simulink model "TRUAV_Dynamics_from_GTRS_trim"  (R2022b)
settings: Solver=ode4  StartTime=0.0  StopTime=3  FixedStep=0.004  RelTol=1e-3
values from neighbouring files (symbols this model uses):
  a_sound = 1116.45    [init_0_GTRS_data_Run_this_file.m]
  alpha_F_rad = alpha_F_deg * (pi/180)    [init_Vetical_2_Table.m]
  alpha_F_rad_table = alpha_F_table * (pi/180)    [init_Fuselage_Aero_Table.m]
  alpha_H_rad = alpha_H_deg * (pi/180)    [init_Horizontal_Table.m]
  alpha_HD_rad = alpha_HD_deg * (pi/180)    [init_Horizontal_C_D_Table.m]
  alpha_r0 = 0    [init_0_GTRS_data_Run_this_file.m]
  alpha_WF_epsilon_M_rad = alpha_WF_deg * pi/180    [init_WingWake_Deflection_Table.m]
  alpha_WS_CL_rad = alpha_WS_CL_deg * (pi/180)    [init_Wing_Slide_Table.m]
  b_w = 32.17    [init_0_GTRS_data_Run_this_file.m]
  beta_F_rad = beta_F_deg * (pi/180)    [init_Vetical_2_Table.m]
  beta_LD_rad_table = beta_LD_table * (pi/180)    [init_Fuselage_Aero_Table.m]
  beta_m_epsilon_M_rad = beta_m_deg * pi/180    [init_WingWake_Deflection_Table.m]
  beta_m_rad_cn = beta_m_deg_cn * pi/180    [init_Wing_Free_Table.m]
  beta_M_rad_table = beta_M_table  * (pi/180)    [init_Fuselage_Aero_Table.m]
  beta_m_S_rad = beta_m_S_deg * (pi/180)    [init_Vetical_2_Table.m]
  beta_m_WS_CL_rad = beta_m_WS_CL_deg * (pi/180)    [init_Wing_Slide_Table.m]
  beta_rad_brk = beta_KBR_rad    [init_Vetical_2_Table.m]
  beta_v_rad = beta_v_deg * (pi/180)    [init_Vetical_1_Table.m]
  beta_vD_rad = beta_vD_deg * (pi/180)    [init_Vetical_1_Table.m]
  beta_WF_Cl_rad = beta_W_deg * (pi/180)    [init_Wing_Free_Table.m]
  beta_WF_CL_rad = beta_CL_deg * (pi/180)    [init_Wing_Free_Table.m]
  beta_YlN_rad_table = beta_YlN_table * (pi/180)    [init_Fuselage_Aero_Table.m]
  c_HW = 3.92    [init_0_GTRS_data_Run_this_file.m]
  C_l_beta_CLwp_table = [ ... (first row only)    [init_Wing_Free_Table.m]
  C_l_beta_pro_CLwp_table = [ ... (first row only)    [init_Wing_Free_Table.m]
  C_L_delta_a_table = [0.00316, 0.00396, 0.00476, 0]    [init_Wing_Free_Table.m]
  C_LHB = -0.00422    [init_0_GTRS_data_Run_this_file.m]
  C_lp_C_LWP = -0.774    [init_0_GTRS_data_Run_this_file.m]
  C_m_wp_table = [ ... (first row only)    [init_Wing_Free_Table.m]
  C_MHA = 0    [init_0_GTRS_data_Run_this_file.m]
  C_MHO = 0    [init_0_GTRS_data_Run_this_file.m]
  c_R = 14/12    (= 1.16666666667)    [init_0_GTRS_data_Run_this_file.m]
  c_w = 5.225    [init_0_GTRS_data_Run_this_file.m]
  C_Y_beta = 0    [init_0_GTRS_data_Run_this_file.m]
  CD0_high_Mach_data = [0.0177, 0.0178, 0.0179, 0.0405]    [init_Wing_Free_Table.m]
  CD_4D_table = zeros(49, 4, 2, 4)    [init_Wing_Slide_Table.m]
  CDH_2D_table = zeros(length(alpha_HD_deg), length(mach_vec))    [init_Horizontal_C_D_Table.m]
  CDV_2D_table = zeros(length(beta_vD_deg), length(mach_vec))    [init_Vetical_1_Table.m]
  CL_4D_table = zeros(49, 4, 2, 4)    [init_Wing_Slide_Table.m]
  CLH_3D_table = zeros(length(alpha_H_deg), length(delta_e_deg), length(mach_vec))    [init_Horizontal_Table.m]
  CYV_3D_table = zeros(length(beta_v_deg), length(delta_r_deg), length(mach_vec))    [init_Vetical_1_Table.m]
  D_alpha_table = [D_part1, D_part2, D_part3, D_part4]    [init_Fuselage_Aero_Table.m]
  D_beta_table = [ fliplr(D_beta_half(2:end)),  D_beta_half]    [init_Fuselage_Aero_Table.m]
  D_ke = 0.24    [init_0_GTRS_data_Run_this_file.m]
  D_Kr = 0.24    [init_0_GTRS_data_Run_this_file.m]    (also in init_Vetical_1_Table.m)
  DBFO = -1.56    [init_0_GTRS_data_Run_this_file.m]
  delta_e_rad = delta_e_deg * (pi/180)    [init_Horizontal_Table.m]
  delta_r_deg = [-20, -15, 0, 15, 20]    [init_Vetical_1_Table.m]
  DLANG = -0.5    [init_0_GTRS_data_Run_this_file.m]
  epsilon_W_table = permute(epsilon_W_3D, [3, 1, 2])    [init_WingWake_Deflection_Table.m]
  flap_rad = flap_deg * (pi/180)    [init_Wing_Free_Table.m]    (also in init_Wing_Slide_Table.m)
  ft2m = 0.3048    [init_0_GTRS_data_Run_this_file.m]
  h_HW = [-0.5838, 0.01158, 0.5967, 0.002547,-2.2519]    [init_0_GTRS_data_Run_this_file.m]
  I_b = 102.5    [init_0_GTRS_data_Run_this_file.m]
  i_H = 0    [init_0_GTRS_data_Run_this_file.m]
  i_v = 0    [init_0_GTRS_data_Run_this_file.m]
  i_w = 0    [init_0_GTRS_data_Run_this_file.m]
  in2ft = 1/12    (= 0.0833333333333)    [init_0_GTRS_data_Run_this_file.m]
  Ixx = 52795    [init_0_GTRS_data_Run_this_file.m]
  Ixz = 1234    [init_0_GTRS_data_Run_this_file.m]
  Iyy = 21360    [init_0_GTRS_data_Run_this_file.m]
  Izz = 66335    [init_0_GTRS_data_Run_this_file.m]
  K1delta_data = [ ... (first row only)    [init_Wing_Free_Table.m]
  K_coeffs = [1.6 0]    [init_0_GTRS_data_Run_this_file.m]
  K_FWDF = -0.0035    [init_0_GTRS_data_Run_this_file.m]
  K_FWO = 1.4    [init_0_GTRS_data_Run_this_file.m]
  K_HNU = 0.8    [init_0_GTRS_data_Run_this_file.m]
  K_vNU = 1    [init_Vetical_1_Table.m]
  KBR_table = KBR_table_full    [init_Vetical_2_Table.m]
  Kn_delta_data = [ ... (first row only)    [init_Wing_Free_Table.m]
  Kno_delta_data = [ ... (first row only)    [init_Wing_Free_Table.m]
  L_alpha_table = [L_part1, L_part2, L_part3, L_part4]    [init_Fuselage_Aero_Table.m]
  L_beta_table = [ fliplr(L_beta_half(2:end)),  L_beta_half]    [init_Fuselage_Aero_Table.m]
  l_beta_table = [l_beta_neg, l_beta_pos]    [init_Fuselage_Aero_Table.m]
  L_n = 4.667    [init_0_GTRS_data_Run_this_file.m]
  lambda_w = -6.5*deg2rad    (= -0.11344640138)    [init_0_GTRS_data_Run_this_file.m]
  LBFO = -7.23    [init_0_GTRS_data_Run_this_file.m]
  LLANG = 0    [init_0_GTRS_data_Run_this_file.m]
  m2ft = 1/ft2m    (= 3.28083989501)    [init_0_GTRS_data_Run_this_file.m]
  M_alpha_table = [M_part1, M_part2, M_part3, M_part4]    [init_Fuselage_Aero_Table.m]
  M_beta_table = [ fliplr(M_beta_half(2:end)), M_beta_half]    [init_Fuselage_Aero_Table.m]
  Mach_brk = [0.2, 0.4, 0.5, 0.6]    [init_Wing_Free_Table.m]
  mach_vec = [0.2, 0.4, 0.5, 0.6]    [init_Horizontal_C_D_Table.m]    (also in init_Horizontal_Table.m; init_Vetical_1_Table.m)
  mass = 403.7    [init_0_GTRS_data_Run_this_file.m]
  mast_rad = mast_deg * pi/180    [init_Wing_Free_Table.m]
  MBFO = 66.5    [init_0_GTRS_data_Run_this_file.m]
  Mn_X_ke = [0 0.2 0.4 0.5 0.6 0.7]    [init_Horizontal_Table.m]
  N_beta_table = [N_beta_neg, N_beta_pos]    [init_Fuselage_Aero_Table.m]
  pos_x_CG = 300    [init_0_GTRS_data_Run_this_file.m]
  pos_x_H = 300    [init_0_GTRS_data_Run_this_file.m]
  pos_x_HW = 560    [init_0_GTRS_data_Run_this_file.m]
  pos_x_Nac = 291.7    [init_0_GTRS_data_Run_this_file.m]
  pos_x_V = 570    [init_0_GTRS_data_Run_this_file.m]
  pos_x_W = 291.7    [init_0_GTRS_data_Run_this_file.m]
  pos_y_CG = 0    [init_0_GTRS_data_Run_this_file.m]
  pos_y_H = 193    [init_0_GTRS_data_Run_this_file.m]
  pos_y_HW = 0    [init_0_GTRS_data_Run_this_file.m]
  pos_y_Nac = 193    [init_0_GTRS_data_Run_this_file.m]
  pos_y_V = 115.69    [init_0_GTRS_data_Run_this_file.m]
  pos_y_W = 96.6    [init_0_GTRS_data_Run_this_file.m]
  pos_z_CG = 81.65    [init_0_GTRS_data_Run_this_file.m]
  pos_z_H = 100    [init_0_GTRS_data_Run_this_file.m]
  pos_z_HW = 103    [init_0_GTRS_data_Run_this_file.m]
  pos_z_Nac = 118    [init_0_GTRS_data_Run_this_file.m]
  pos_z_V = 77    [init_0_GTRS_data_Run_this_file.m]
  pos_z_W = 96    [init_0_GTRS_data_Run_this_file.m]
  R = 12.5    [init_0_GTRS_data_Run_this_file.m]
  rho = 0.002376    [init_0_GTRS_data_Run_this_file.m]
  s_HW = 50.25    [init_0_GTRS_data_Run_this_file.m]
  S_max = 56    [init_0_GTRS_data_Run_this_file.m]
  S_v = 20.25    [init_0_GTRS_data_Run_this_file.m]
  S_w = 181    [init_0_GTRS_data_Run_this_file.m]
  Sidewash_4D = zeros(length(alpha_F_deg), length(beta_F_deg), length(beta_m_S_deg), length(delta_F_S_deg))    [init_Vetical_2_Table.m]
  slugft2kgm = 1.35582    [init_0_GTRS_data_Run_this_file.m]
  tau_e = 0.518    [init_0_GTRS_data_Run_this_file.m]
  tau_r = 0.27    [init_0_GTRS_data_Run_this_file.m]    (also in init_Vetical_1_Table.m)
  theta_0_R = 0.750    (= 0.75)    [init_0_GTRS_data_Run_this_file.m]
  theta_0_W = 1.187    [init_0_GTRS_data_Run_this_file.m]
  theta_twist = -41*deg2rad    (= -0.715584993318)    [init_0_GTRS_data_Run_this_file.m]
  u_max = 1181/12    (= 98.4166666667)    [init_0_GTRS_data_Run_this_file.m]
  ... (+3 more)
undefined symbols (not defined in the file or in its folder): beta_m_rad, F, Light, MIL, sigbuilder_block, tilt_cmd
libraries: simulink x2, sharedtransform x2, aerolibasang x2, aerolibwind2 x1
(part 2 of 4)

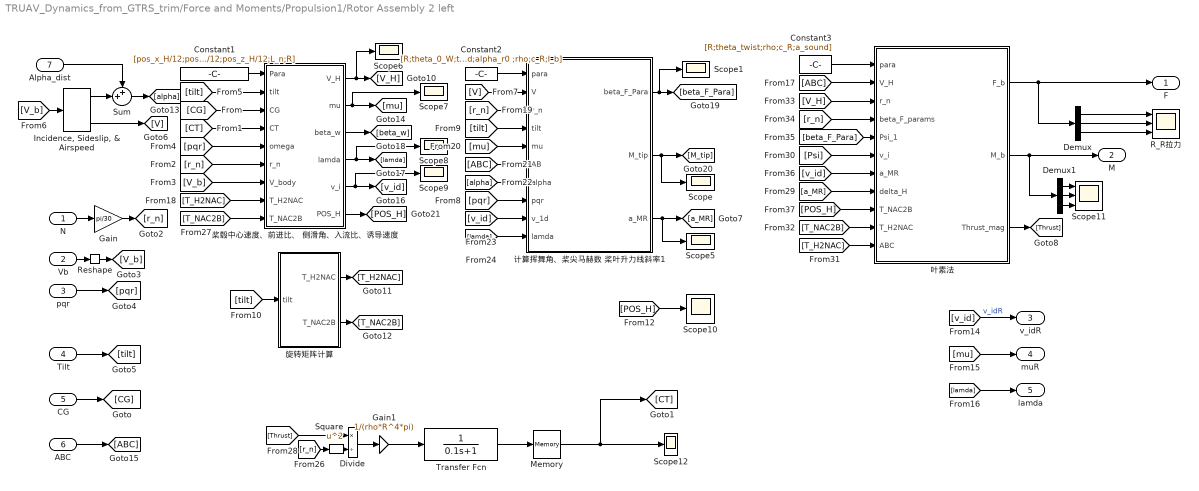
== system TRUAV_Dynamics_from_GTRS_trim/Force and Moments/Propulsion1/Rotor Assembly 2 left ==
  N : Inport
  Vb : Inport  Port=2
  pqr : Inport  Port=3
  Tilt : Inport  Port=4
  CG : Inport  Port=5
  ABC : Inport  Port=6
  Alpha_dist : Inport  Port=7
  Constant1 : Constant  Value=[pos_x_H/12;pos_y_H/12;pos_z_H/12;L_n;R]
  Constant2 : Constant  Value=[R;theta_0_W;theta_0_R;theta_twist;a_sound;alpha_r0 ;rho;c_R;I_b]
  Constant3 : Constant  Value=[R;theta_twist;rho;c_R;a_sound]
  Demux : Demux  Outputs=3
  Demux1 : Demux  Outputs=3
  Divide : Product  Inputs=*/
  Gain : Gain  Gain=pi/30
  Gain1 : Gain  Gain=1/(rho*R^4*pi)
  "Incidence, Sideslip, & Airspeed" : aerolibasang/Incidence, Sideslip, & Airspeed
  Memory : Memory  InitialCondition=0.02
  R_R拉力 : Scope  NumInputPorts=3
  Reshape : Reshape  OutputDimensionality=Column vector (2-D)
  Scope{,1,5..10,12} (9 alike) : Scope
  Scope11 : Scope  NumInputPorts=3
  Square : Math  Operator=square
  Sum : Sum  Inputs=++|
  Transfer Fcn : TransferFcn  Denominator=[0.1 1]
  叶素法 : MATLAB Function  TreatAsAtomicUnit=on
  旋转矩阵计算 : MATLAB Function  TreatAsAtomicUnit=on
  桨毂中心速度、前进比、 侧滑角、入流比、诱导速度 : MATLAB Function  TreatAsAtomicUnit=on
  计算挥舞角、桨尖马赫数 桨叶升力线斜率1 : MATLAB Function  TreatAsAtomicUnit=on
  F : Outport
  M : Outport  Port=2
  v_idR : Outport  Port=3
  muR : Outport  Port=4
  lamda : Outport  Port=5
  wires:
  Demux1/3 -> Scope11/3
  Demux1/2 -> Scope11/2
  Demux1/1 -> Scope11/1
  Demux/3 -> R_R拉力/3
  Demux/2 -> R_R拉力/2
  Demux/1 -> R_R拉力/1
  [Psi] -> 叶素法/6(v_i)
  桨毂中心速度、前进比、 侧滑角、入流比、诱导速度/3(beta_w) -> [beta_w]
  Reshape/1 -> [V_b]
  [POS_H] -> Scope10/1
  [T_NAC2B] -> 桨毂中心速度、前进比、 侧滑角、入流比、诱导速度/9(T_NAC2B)
  Gain/1 -> [r_n]
  pqr/1 -> [pqr]
  N/1 -> Gain/1
  Constant1/1 -> 桨毂中心速度、前进比、 侧滑角、入流比、诱导速度/1(Para)
  CG/1 -> [CG]
  [CG] -> 桨毂中心速度、前进比、 侧滑角、入流比、诱导速度/3(CG)
  [CT] -> 桨毂中心速度、前进比、 侧滑角、入流比、诱导速度/4(CT)
  [r_n] -> 桨毂中心速度、前进比、 侧滑角、入流比、诱导速度/6(r_n)
  Vb/1 -> Reshape/1
  [V_b] -> 桨毂中心速度、前进比、 侧滑角、入流比、诱导速度/7(V_body)
  [pqr] -> 桨毂中心速度、前进比、 侧滑角、入流比、诱导速度/5(omega)
  Tilt/1 -> [tilt]
  [tilt] -> 桨毂中心速度、前进比、 侧滑角、入流比、诱导速度/2(tilt)
  [V] -> 计算挥舞角、桨尖马赫数 桨叶升力线斜率1/2(V)
  [tilt] -> 计算挥舞角、桨尖马赫数 桨叶升力线斜率1/4(tilt)
  Constant2/1 -> 计算挥舞角、桨尖马赫数 桨叶升力线斜率1/1(para)
  计算挥舞角、桨尖马赫数 桨叶升力线斜率1/3(a_MR) -> [a_MR], Scope5/1
  [pqr] -> 计算挥舞角、桨尖马赫数 桨叶升力线斜率1/8(pqr)
  桨毂中心速度、前进比、 侧滑角、入流比、诱导速度/1(V_H) -> [V_H], Scope6/1
  [tilt] -> 旋转矩阵计算/1(tilt)
  旋转矩阵计算/1(T_H2NAC) -> [T_H2NAC]
  旋转矩阵计算/2(T_NAC2B) -> [T_NAC2B]
  [T_H2NAC] -> 桨毂中心速度、前进比、 侧滑角、入流比、诱导速度/8(T_H2NAC)
  桨毂中心速度、前进比、 侧滑角、入流比、诱导速度/2(mu) -> [mu], Scope7/1
  [r_n] -> 计算挥舞角、桨尖马赫数 桨叶升力线斜率1/3(r_n)
  [mu] -> 计算挥舞角、桨尖马赫数 桨叶升力线斜率1/5(mu)
  [ABC] -> 计算挥舞角、桨尖马赫数 桨叶升力线斜率1/6(AB)
  [alpha] -> 计算挥舞角、桨尖马赫数 桨叶升力线斜率1/7(alpha)
  桨毂中心速度、前进比、 侧滑角、入流比、诱导速度/5(v_i) -> [v_id], Scope9/1
  [v_id] -> 计算挥舞角、桨尖马赫数 桨叶升力线斜率1/9(v_1d)
  桨毂中心速度、前进比、 侧滑角、入流比、诱导速度/4(lamda) -> [lamda], Scope8/1
  [lamda] -> 计算挥舞角、桨尖马赫数 桨叶升力线斜率1/10(lamda)
  计算挥舞角、桨尖马赫数 桨叶升力线斜率1/1(beta_F_Para) -> [beta_F_Para], Scope1/1
  计算挥舞角、桨尖马赫数 桨叶升力线斜率1/2(M_tip) -> [M_tip], Scope/1
  桨毂中心速度、前进比、 侧滑角、入流比、诱导速度/6(POS_H) -> [POS_H]
  ABC/1 -> [ABC]
  [POS_H] -> 叶素法/9(T_NAC2B)
  [v_id] -> 叶素法/7(a_MR)
  [beta_F_Para] -> 叶素法/5(Psi_1)
  [r_n] -> 叶素法/4(beta_F_params)
  [V_H] -> 叶素法/3(r_n)
  Constant3/1 -> 叶素法/1(para)
  [a_MR] -> 叶素法/8(delta_H)
  [T_NAC2B] -> 叶素法/10(T_H2NAC)
  [T_H2NAC] -> 叶素法/11(ABC)
  [v_id] -> v_idR/1  "v_idR"
  [lamda] -> lamda/1
  [mu] -> muR/1
  [ABC] -> 叶素法/2(V_H)
  叶素法/1(F_b) -> F/1, Demux/1
  [r_n] -> Square/1
  Transfer Fcn/1 -> Memory/1
  [Thrust] -> Divide/1
  Divide/1 -> Gain1/1
  Square/1 -> Divide/2
  Gain1/1 -> Transfer Fcn/1
  叶素法/3(Thrust_mag) -> [Thrust]
  Memory/1 -> [CT], Scope12/1
  [V_b] -> "Incidence, Sideslip, & Airspeed"/1
  Alpha_dist/1 -> Sum/1
  Sum/1 -> [alpha]
  "Incidence, Sideslip, & Airspeed"/1 -> Sum/2
  "Incidence, Sideslip, & Airspeed"/3 -> [V]
  叶素法/2(M_b) -> Demux1/1, M/1

== system TRUAV_Dynamics_from_GTRS_trim/Force and Moments/Propulsion1/Tilt Servo Dynamics ==
  TiltA : Inport
  Tilt1 : Outport
  wires:
  TiltA/1 -> Tilt1/1  "Tilt1"

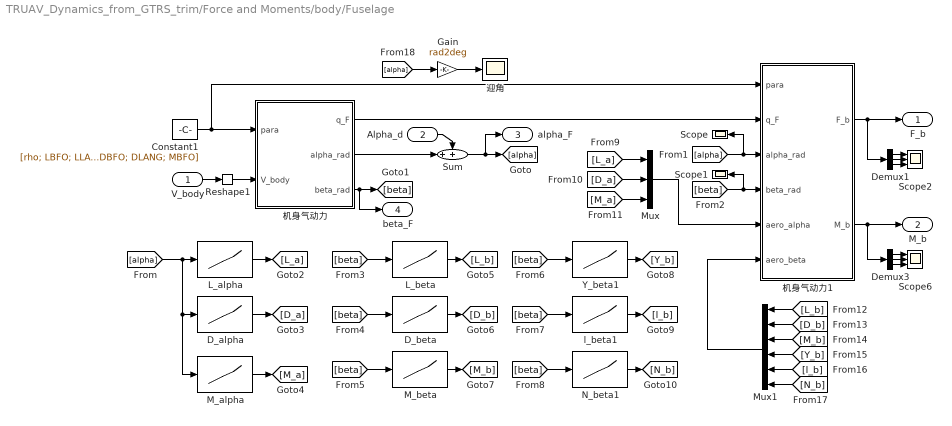
== system TRUAV_Dynamics_from_GTRS_trim/Force and Moments/body/Fuselage ==
  V_body : Inport
  Alpha_d : Inport  Port=2
  Constant1 : Constant  Value=[rho; LBFO; LLANG; DBFO; DLANG; MBFO]
  D_alpha : Lookup_n-D  NumberOfTableDimensions=1  LookupTableObject=''  BreakpointsForDimension1=alpha_F_rad_table  BreakpointsForDimension1FirstPoint=10  BreakpointsForDimension2FirstPoint=10  BreakpointsForDimension1Spacing=12  BreakpointsForDimension2Spacing=12  Table=D_alpha_table  DiagnosticForOutOfRangeInput=Error  InternalRulePriority=Speed  RndMeth=Simplest
  D_beta : Lookup_n-D  NumberOfTableDimensions=1  LookupTableObject=''  BreakpointsForDimension1=beta_LD_rad_table  BreakpointsForDimension1FirstPoint=10  BreakpointsForDimension2FirstPoint=10  BreakpointsForDimension1Spacing=12  BreakpointsForDimension2Spacing=12  Table=D_beta_table  DiagnosticForOutOfRangeInput=Error  InternalRulePriority=Speed  RndMeth=Simplest
  Demux1 : Demux  Outputs=3
  Demux3 : Demux  Outputs=3
  Gain : Gain  Gain=rad2deg
  L_alpha : Lookup_n-D  NumberOfTableDimensions=1  LookupTableObject=''  BreakpointsForDimension1=alpha_F_rad_table  BreakpointsForDimension1FirstPoint=10  BreakpointsForDimension2FirstPoint=10  BreakpointsForDimension1Spacing=12  BreakpointsForDimension2Spacing=12  Table=L_alpha_table  DiagnosticForOutOfRangeInput=Error  InternalRulePriority=Speed  RndMeth=Simplest
  L_beta : Lookup_n-D  NumberOfTableDimensions=1  LookupTableObject=''  BreakpointsForDimension1=beta_LD_rad_table  BreakpointsForDimension1FirstPoint=10  BreakpointsForDimension2FirstPoint=10  BreakpointsForDimension1Spacing=12  BreakpointsForDimension2Spacing=12  Table=L_beta_table  DiagnosticForOutOfRangeInput=Error  InternalRulePriority=Speed  RndMeth=Simplest
  M_alpha : Lookup_n-D  NumberOfTableDimensions=1  LookupTableObject=''  BreakpointsForDimension1=alpha_F_rad_table  BreakpointsForDimension1FirstPoint=10  BreakpointsForDimension2FirstPoint=10  BreakpointsForDimension1Spacing=12  BreakpointsForDimension2Spacing=12  IndexSearchMethod=Linear search  Table=M_alpha_table  DiagnosticForOutOfRangeInput=Error  InternalRulePriority=Speed  RndMeth=Simplest
  M_beta : Lookup_n-D  NumberOfTableDimensions=1  LookupTableObject=''  BreakpointsForDimension1=beta_M_rad_table  BreakpointsForDimension1FirstPoint=10  BreakpointsForDimension2FirstPoint=10  BreakpointsForDimension1Spacing=12  BreakpointsForDimension2Spacing=12  Table=M_beta_table  DiagnosticForOutOfRangeInput=Error  InternalRulePriority=Speed  RndMeth=Simplest
  Mux : Mux  Inputs=3
  Mux1 : Mux  Inputs=6
  N_beta1 : Lookup_n-D  NumberOfTableDimensions=1  LookupTableObject=''  BreakpointsForDimension1=beta_YlN_rad_table  BreakpointsForDimension1FirstPoint=10  BreakpointsForDimension2FirstPoint=10  BreakpointsForDimension1Spacing=12  BreakpointsForDimension2Spacing=12  Table=N_beta_table  DiagnosticForOutOfRangeInput=Error  InternalRulePriority=Speed  RndMeth=Simplest
  Reshape1 : Reshape  OutputDimensionality=Column vector (2-D)
  Scope : Scope
  Scope1 : Scope
  Scope2 : Scope  NumInputPorts=3
  Scope6 : Scope  NumInputPorts=3
  Sum : Sum  Inputs=++|
  Y_beta1 : Lookup_n-D  NumberOfTableDimensions=1  LookupTableObject=''  BreakpointsForDimension1=beta_YlN_rad_table  BreakpointsForDimension1FirstPoint=10  BreakpointsForDimension2FirstPoint=10  BreakpointsForDimension1Spacing=12  BreakpointsForDimension2Spacing=12  Table=Y_beta_table  DiagnosticForOutOfRangeInput=Error  InternalRulePriority=Speed  RndMeth=Simplest
  l_beta1 : Lookup_n-D  NumberOfTableDimensions=1  LookupTableObject=''  BreakpointsForDimension1=beta_YlN_rad_table  BreakpointsForDimension1FirstPoint=10  BreakpointsForDimension2FirstPoint=10  BreakpointsForDimension1Spacing=12  BreakpointsForDimension2Spacing=12  Table=l_beta_table  DiagnosticForOutOfRangeInput=Error  InternalRulePriority=Speed  RndMeth=Simplest
  机身气动力 : MATLAB Function  TreatAsAtomicUnit=on
  机身气动力1 : MATLAB Function  TreatAsAtomicUnit=on
  迎角 : Scope
  F_b : Outport
  M_b : Outport  Port=2
  alpha_F : Outport  Port=3
  beta_F : Outport  Port=4
  wires:
  Constant1/1 -> 机身气动力1/1(para), 机身气动力/1(para)
  V_body/1 -> Reshape1/1
  机身气动力/1(q_F) -> 机身气动力1/2(q_F)
  Sum/1 -> alpha_F/1, [alpha]
  机身气动力/3(beta_rad) -> beta_F/1, [beta]
  [alpha] -> M_alpha/1, D_alpha/1, L_alpha/1
  [alpha] -> Scope/1, 机身气动力1/3(alpha_rad)
  [beta] -> Scope1/1, 机身气动力1/4(beta_rad)
  L_alpha/1 -> [L_a]
  D_alpha/1 -> [D_a]
  M_alpha/1 -> [M_a]
  [beta] -> L_beta/1
  [beta] -> D_beta/1
  L_beta/1 -> [L_b]
  D_beta/1 -> [D_b]
  [beta] -> M_beta/1
  M_beta/1 -> [M_b]
  机身气动力1/2(M_b) -> Demux3/1, M_b/1
  N_beta1/1 -> [N_b]
  [beta] -> N_beta1/1
  l_beta1/1 -> [l_b]
  Y_beta1/1 -> [Y_b]
  [beta] -> l_beta1/1
  [beta] -> Y_beta1/1
  [D_a] -> Mux/2
  [L_a] -> Mux/1
  [M_a] -> Mux/3
  [l_b] -> Mux1/5
  [N_b] -> Mux1/6
  [Y_b] -> Mux1/4
  [M_b] -> Mux1/3
  [D_b] -> Mux1/2
  [L_b] -> Mux1/1
  Mux/1 -> 机身气动力1/5(aero_alpha)
  Mux1/1 -> 机身气动力1/6(aero_beta)
  Reshape1/1 -> 机身气动力/2(V_body)
  Demux3/3 -> Scope6/3
  Demux3/2 -> Scope6/2
  Demux3/1 -> Scope6/1
  Demux1/1 -> Scope2/1
  Demux1/2 -> Scope2/2
  Demux1/3 -> Scope2/3
  机身气动力1/1(F_b) -> Demux1/1, F_b/1
  机身气动力/2(alpha_rad) -> Sum/2
  Alpha_d/1 -> Sum/1
  Gain/1 -> 迎角/1
  [alpha] -> Gain/1

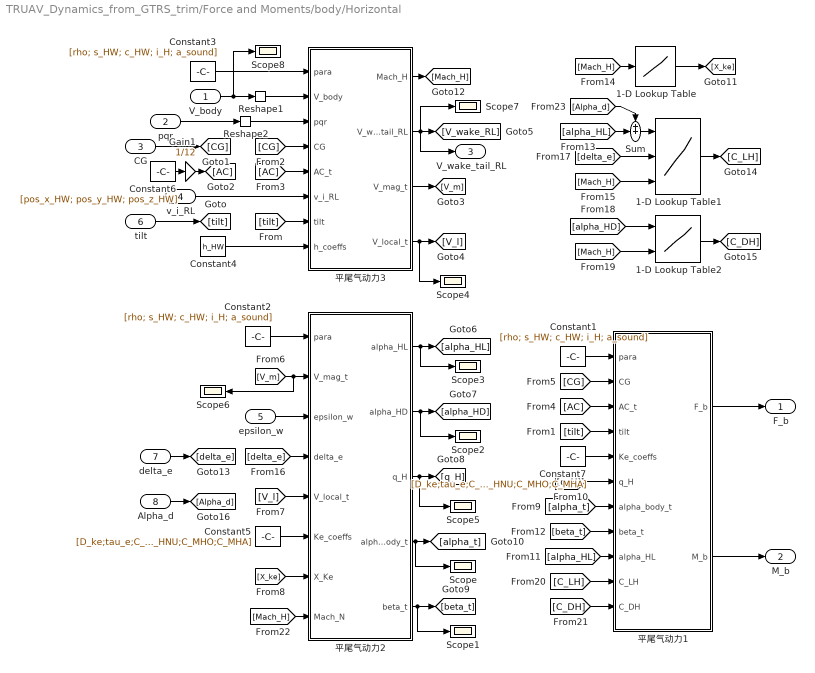
== system TRUAV_Dynamics_from_GTRS_trim/Force and Moments/body/Horizontal ==
  V_body : Inport
  pqr : Inport  Port=2
  CG : Inport  Port=3
  v_i_RL : Inport  Port=4
  epsilon_w : Inport  Port=5
  tilt : Inport  Port=6
  delta_e : Inport  Port=7
  Alpha_d : Inport  Port=8
  1-D Lookup Table : Lookup_n-D  NumberOfTableDimensions=1  BreakpointsForDimension1=Mn_X_ke  Table=X_Ke_table  InternalRulePriority=Speed  RndMeth=Simplest
  1-D Lookup Table1 : Lookup_n-D  NumberOfTableDimensions=3  BreakpointsForDimension1=alpha_H_rad  BreakpointsForDimension2=delta_e_rad  BreakpointsForDimension3=mach_vec  Table=CLH_3D_table  InternalRulePriority=Speed  RndMeth=Simplest
      settings: InputPortMap=u0,u1,u2
  1-D Lookup Table2 : Lookup_n-D  BreakpointsForDimension1=alpha_HD_rad  BreakpointsForDimension2=mach_vec  Table=CDH_2D_table  InternalRulePriority=Speed  RndMeth=Simplest
      settings: InputPortMap=u0,u1
  Constant1 : Constant  Value=[rho; s_HW; c_HW; i_H; a_sound]
  Constant2 : Constant  Value=[rho; s_HW; c_HW; i_H; a_sound]
  Constant3 : Constant  Value=[rho; s_HW; c_HW; i_H; a_sound]
  Constant4 : Constant  Value=h_HW
  Constant5 : Constant  Value=[D_ke;tau_e;C_LHB;K_HNU;C_MHO;C_MHA]
  Constant6 : Constant  Value=[pos_x_HW; pos_y_HW; pos_z_HW]
  Constant7 : Constant  Value=[D_ke;tau_e;C_LHB;K_HNU;C_MHO;C_MHA]
  Gain1 : Gain  Gain=1/12
  Reshape1 : Reshape  OutputDimensionality=Column vector (2-D)
  Reshape2 : Reshape  OutputDimensionality=Column vector (2-D)
  Scope{,1..8} (9 alike) : Scope
  Sum : Sum  Inputs=++|
  平尾气动力1 : MATLAB Function  TreatAsAtomicUnit=on
  平尾气动力2 : MATLAB Function  TreatAsAtomicUnit=on
  平尾气动力3 : MATLAB Function  TreatAsAtomicUnit=on
  F_b : Outport
  M_b : Outport  Port=2
  V_wake_tail_RL : Outport  Port=3
  wires:
  Constant6/1 -> Gain1/1
  v_i_RL/1 -> 平尾气动力3/6(v_i_RL)
  Constant4/1 -> 平尾气动力3/8(h_coeffs)
  CG/1 -> [CG]
  V_body/1 -> Scope8/1, Reshape1/1
  pqr/1 -> Reshape2/1
  Constant3/1 -> 平尾气动力3/1(para)
  Constant2/1 -> 平尾气动力2/1(para)
  epsilon_w/1 -> 平尾气动力2/3(epsilon_w)
  tilt/1 -> [tilt]
  [tilt] -> 平尾气动力3/7(tilt)
  [tilt] -> 平尾气动力1/4(tilt)
  [CG] -> 平尾气动力3/4(CG)
  Gain1/1 -> [AC]
  [AC] -> 平尾气动力3/5(AC_t)
  [AC] -> 平尾气动力1/3(AC_t)
  [CG] -> 平尾气动力1/2(CG)
  Constant1/1 -> 平尾气动力1/1(para)
  平尾气动力3/3(V_mag_t) -> [V_m]
  [V_m] -> Scope6/1, 平尾气动力2/2(V_mag_t)
  平尾气动力3/4(V_local_t) -> Scope4/1, [V_l]
  [V_l] -> 平尾气动力2/5(V_local_t)
  Constant5/1 -> 平尾气动力2/6(Ke_coeffs)
  Constant7/1 -> 平尾气动力1/5(Ke_coeffs)
  平尾气动力3/2(V_wake_tail_RL) -> Scope7/1, V_wake_tail_RL/1, [V_wake_RL]
  平尾气动力2/1(alpha_HL) -> Scope3/1, [alpha_HL]
  平尾气动力2/2(alpha_HD) -> Scope2/1, [alpha_HD]
  平尾气动力2/3(q_H) -> Scope5/1, [q_H]
  平尾气动力2/5(beta_t) -> Scope1/1, [beta_t]
  平尾气动力2/4(alpha_body_t) -> Scope/1, [alpha_t]
  [alpha_t] -> 平尾气动力1/7(alpha_body_t)
  [q_H] -> 平尾气动力1/6(q_H)
  [alpha_HL] -> 平尾气动力1/9(alpha_HL)
  [beta_t] -> 平尾气动力1/8(beta_t)
  平尾气动力1/1(F_b) -> F_b/1
  平尾气动力1/2(M_b) -> M_b/1
  1-D Lookup Table/1 -> [X_ke]
  [X_ke] -> 平尾气动力2/7(X_Ke)
  平尾气动力3/1(Mach_H) -> [Mach_H]
  [Mach_H] -> 1-D Lookup Table/1
  delta_e/1 -> [delta_e]
  [delta_e] -> 平尾气动力2/4(delta_e)
  [Mach_H] -> 1-D Lookup Table2/2
  [alpha_HD] -> 1-D Lookup Table2/1
  [C_LH] -> 平尾气动力1/10(C_LH)
  [C_DH] -> 平尾气动力1/11(C_DH)
  1-D Lookup Table1/1 -> [C_LH]
  1-D Lookup Table2/1 -> [C_DH]
  [Mach_H] -> 1-D Lookup Table1/3
  [delta_e] -> 1-D Lookup Table1/2
  [Mach_H] -> 平尾气动力2/8(Mach_N)
  Reshape1/1 -> 平尾气动力3/2(V_body)
  Reshape2/1 -> 平尾气动力3/3(pqr)
  Alpha_d/1 -> [Alpha_d]
  Sum/1 -> 1-D Lookup Table1/1
  [alpha_HL] -> Sum/2
  [Alpha_d] -> Sum/1

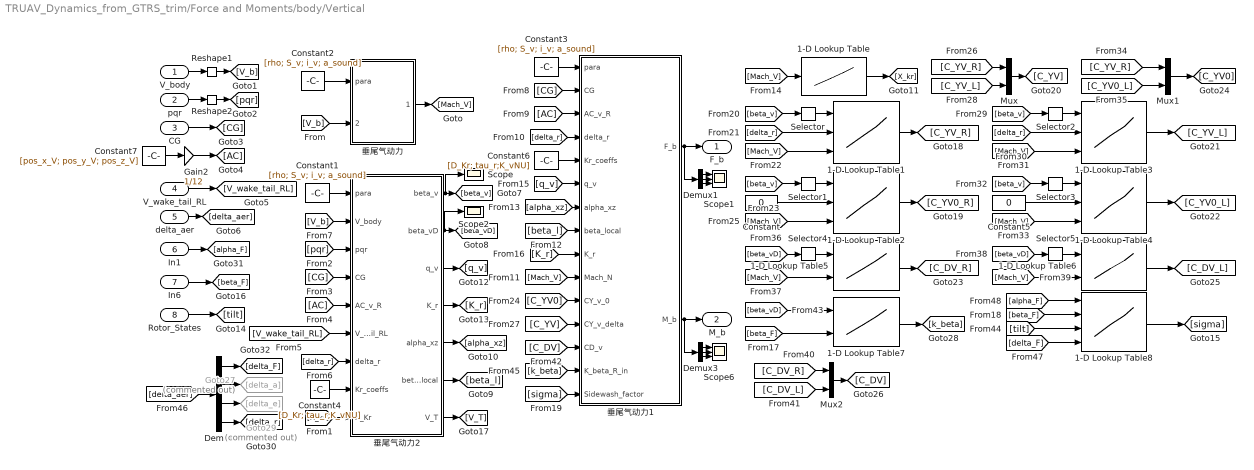
== system TRUAV_Dynamics_from_GTRS_trim/Force and Moments/body/Vertical ==
  V_body : Inport
  pqr : Inport  Port=2
  CG : Inport  Port=3
  V_wake_tail_RL : Inport  Port=4
  delta_aer : Inport  Port=5
  In1 : Inport  Port=6
  In6 : Inport  Port=7
  Rotor_States : Inport  Port=8
  1-D Lookup Table : Lookup_n-D  NumberOfTableDimensions=1  BreakpointsForDimension1=Mn_X_ke  Table=X_Ke_table  InternalRulePriority=Speed  RndMeth=Simplest
  1-D Lookup Table{1..4} (4 alike) : Lookup_n-D  NumberOfTableDimensions=3  BreakpointsForDimension1=beta_v_rad  BreakpointsForDimension2=delta_r_deg  BreakpointsForDimension3=mach_vec  Table=CYV_3D_table  InternalRulePriority=Speed  RndMeth=Simplest
      settings: InputPortMap=u0,u1,u2
  1-D Lookup Table5 : Lookup_n-D  BreakpointsForDimension1=beta_vD_rad  BreakpointsForDimension2=mach_vec  BreakpointsForDimension3=mach_vec  Table=CDV_2D_table  InternalRulePriority=Speed  RndMeth=Simplest
      settings: InputPortMap=u0,u1
  1-D Lookup Table6 : Lookup_n-D  BreakpointsForDimension1=beta_vD_rad  BreakpointsForDimension2=mach_vec  BreakpointsForDimension3=mach_vec  Table=CDV_2D_table  InternalRulePriority=Speed  RndMeth=Simplest
      settings: InputPortMap=u0,u1
  1-D Lookup Table7 : Lookup_n-D  BreakpointsForDimension1=VT_fts_brk  BreakpointsForDimension2=beta_rad_brk  BreakpointsForDimension3=mach_vec  Table=KBR_table  InternalRulePriority=Speed  RndMeth=Simplest
      settings: InputPortMap=u0,u1
  1-D Lookup Table8 : Lookup_n-D  NumberOfTableDimensions=4  BreakpointsForDimension1=alpha_F_rad  BreakpointsForDimension2=beta_F_rad  BreakpointsForDimension3=beta_m_S_rad  BreakpointsForDimension4=delta_F_S_rad  Table=Sidewash_4D  InternalRulePriority=Speed  RndMeth=Simplest
      settings: InputPortMap=u0,u1,u2,u3
  Constant : Constant  Value=0
  Constant1 : Constant  Value=[rho; S_v; i_v; a_sound]
  Constant2 : Constant  Value=[rho; S_v; i_v; a_sound]
  Constant3 : Constant  Value=[rho; S_v; i_v; a_sound]
  Constant4 : Constant  Value=[D_Kr; tau_r;K_vNU]
  Constant5 : Constant  Value=0
  Constant6 : Constant  Value=[D_Kr; tau_r;K_vNU]
  Constant7 : Constant  Value=[pos_x_V; pos_y_V; pos_z_V]
  Demux : Demux
  Demux1 : Demux  Outputs=3
  Demux3 : Demux  Outputs=3
  Gain2 : Gain  Gain=1/12
  Goto27 : Goto  Commented=on  GotoTag=delta_a
  Goto29 : Goto  Commented=on  GotoTag=delta_e
  Mux : Mux  Inputs=2
  Mux1 : Mux  Inputs=2
  Mux2 : Mux  Inputs=2
  Reshape1 : Reshape  OutputDimensionality=Column vector (2-D)
  Reshape2 : Reshape  OutputDimensionality=Column vector (2-D)
  Scope : Scope
  Scope1 : Scope  NumInputPorts=3
  Scope2 : Scope
  Scope6 : Scope  NumInputPorts=3
  Selector : Selector  InputPortWidth=2  IndexOptions=Index vector (dialog)  Indices=[1]  OutputSizes=1
  Selector1 : Selector  InputPortWidth=2  IndexOptions=Index vector (dialog)  Indices=[1]  OutputSizes=1
  Selector2 : Selector  InputPortWidth=2  IndexOptions=Index vector (dialog)  Indices=[2]  OutputSizes=1
  Selector3 : Selector  InputPortWidth=2  IndexOptions=Index vector (dialog)  Indices=[2]  OutputSizes=1
  Selector4 : Selector  InputPortWidth=2  IndexOptions=Index vector (dialog)  Indices=[1]  OutputSizes=1
  Selector5 : Selector  InputPortWidth=2  IndexOptions=Index vector (dialog)  Indices=[2]  OutputSizes=1
  垂尾气动力 : MATLAB Function  TreatAsAtomicUnit=on
  垂尾气动力1 : MATLAB Function  TreatAsAtomicUnit=on
  垂尾气动力2 : MATLAB Function  TreatAsAtomicUnit=on
  F_b : Outport
  M_b : Outport  Port=2
  wires:
  Constant7/1 -> Gain2/1
  V_body/1 -> Reshape1/1
  Constant2/1 -> 垂尾气动力/1(para)
  [Mach_V] -> 1-D Lookup Table/1
  1-D Lookup Table/1 -> [X_kr]
  Constant1/1 -> 垂尾气动力2/1(para)
  Constant3/1 -> 垂尾气动力1/1(para)
  [V_b] -> 垂尾气动力/2(V_body)
  垂尾气动力/1(Mach_N) -> [Mach_V]
  [X_kr] -> 垂尾气动力2/9(X_Kr)
  pqr/1 -> Reshape2/1
  [pqr] -> 垂尾气动力2/3(pqr)
  CG/1 -> [CG]
  [CG] -> 垂尾气动力2/4(CG)
  Gain2/1 -> [AC]
  [AC] -> 垂尾气动力2/5(AC_v_R)
  V_wake_tail_RL/1 -> [V_wake_tail_RL]
  [V_wake_tail_RL] -> 垂尾气动力2/6(V_wake_tail_RL)
  delta_aer/1 -> [delta_aer]
  [delta_r] -> 垂尾气动力2/7(delta_r)
  [V_b] -> 垂尾气动力2/2(V_body)
  [CG] -> 垂尾气动力1/2(CG)
  [AC] -> 垂尾气动力1/3(AC_v_R)
  [delta_r] -> 垂尾气动力1/4(delta_r)
  垂尾气动力2/1(beta_v) -> Scope/1, [beta_v]
  垂尾气动力2/2(beta_vD) -> Scope2/1, [beta_vD]
  [Mach_V] -> 垂尾气动力1/10(Mach_N)
  垂尾气动力2/6(beta_local) -> [beta_l]
  [beta_l] -> 垂尾气动力1/8(beta_local)
  垂尾气动力2/5(alpha_xz) -> [alpha_xz]
  [alpha_xz] -> 垂尾气动力1/7(alpha_xz)
  垂尾气动力2/3(q_v) -> [q_v]
  [q_v] -> 垂尾气动力1/6(q_v)
  垂尾气动力2/4(K_r) -> [K_r]
  [K_r] -> 垂尾气动力1/9(K_r)
  Constant4/1 -> 垂尾气动力2/8(Kr_coeffs)
  Constant6/1 -> 垂尾气动力1/5(Kr_coeffs)
  [sigma] -> 垂尾气动力1/15(Sidewash_factor)
  垂尾气动力1/1(F_b) -> F_b/1, Demux1/1
  垂尾气动力1/2(M_b) -> Demux3/1, M_b/1
  In6/1 -> [beta_F]
  垂尾气动力2/7(V_T) -> [V_T]
  [beta_v] -> Selector/1
  [Mach_V] -> 1-D Lookup Table1/3
  1-D Lookup Table1/1 -> [C_YV_R]
  1-D Lookup Table2/1 -> [C_YV0_R]
  [Mach_V] -> 1-D Lookup Table2/3
  Constant/1 -> 1-D Lookup Table2/2
  [beta_v] -> Selector1/1
  [C_YV0] -> 垂尾气动力1/11(CY_v_0)
  Selector/1 -> 1-D Lookup Table1/1
  [delta_r] -> 1-D Lookup Table1/2
  Selector1/1 -> 1-D Lookup Table2/1
  [C_YV_R] -> Mux/1
  [C_YV_L] -> Mux/2
  Mux/1 -> [C_YV]
  [C_YV] -> 垂尾气动力1/12(CY_v_delta)
  [delta_r] -> 1-D Lookup Table3/2
  Selector2/1 -> 1-D Lookup Table3/1
  1-D Lookup Table3/1 -> [C_YV_L]
  [Mach_V] -> 1-D Lookup Table3/3
  [beta_v] -> Selector2/1
  Selector3/1 -> 1-D Lookup Table4/1
  [beta_v] -> Selector3/1
  Constant5/1 -> 1-D Lookup Table4/2
  [Mach_V] -> 1-D Lookup Table4/3
  1-D Lookup Table4/1 -> [C_YV0_L]
  Mux1/1 -> [C_YV0]
  [C_YV_R] -> Mux1/1
  [C_YV0_L] -> Mux1/2
  Selector4/1 -> 1-D Lookup Table5/1
  [beta_vD] -> Selector4/1
  [Mach_V] -> 1-D Lookup Table5/2
  1-D Lookup Table5/1 -> [C_DV_R]
  1-D Lookup Table6/1 -> [C_DV_L]
  [Mach_V] -> 1-D Lookup Table6/2
  [beta_vD] -> Selector5/1
  Selector5/1 -> 1-D Lookup Table6/1
  Mux2/1 -> [C_DV]
  [C_DV_L] -> Mux2/2
  [C_DV_R] -> Mux2/1
  [C_DV] -> 垂尾气动力1/13(CD_v)
  1-D Lookup Table7/1 -> [k_beta]
  [beta_F] -> 1-D Lookup Table7/2
  [beta_vD] -> 1-D Lookup Table7/1
  [k_beta] -> 垂尾气动力1/14(K_beta_R_in)
  1-D Lookup Table8/1 -> [sigma]
  [beta_F] -> 1-D Lookup Table8/2
  Rotor_States/1 -> [tilt]
  [tilt] -> 1-D Lookup Table8/3
  [delta_F] -> 1-D Lookup Table8/4
  In1/1 -> [alpha_F]
  [alpha_F] -> 1-D Lookup Table8/1
  Demux/4 -> [delta_r]
  Demux/2 -> Goto27/1
  [delta_aer] -> Demux/1
  Demux/1 -> [delta_F]
  Demux/3 -> Goto29/1
  Reshape1/1 -> [V_b]
  Reshape2/1 -> [pqr]
  Demux3/1 -> Scope6/1
  Demux3/3 -> Scope6/3
  Demux3/2 -> Scope6/2
  Demux1/1 -> Scope1/1
  Demux1/3 -> Scope1/3
  Demux1/2 -> Scope1/2

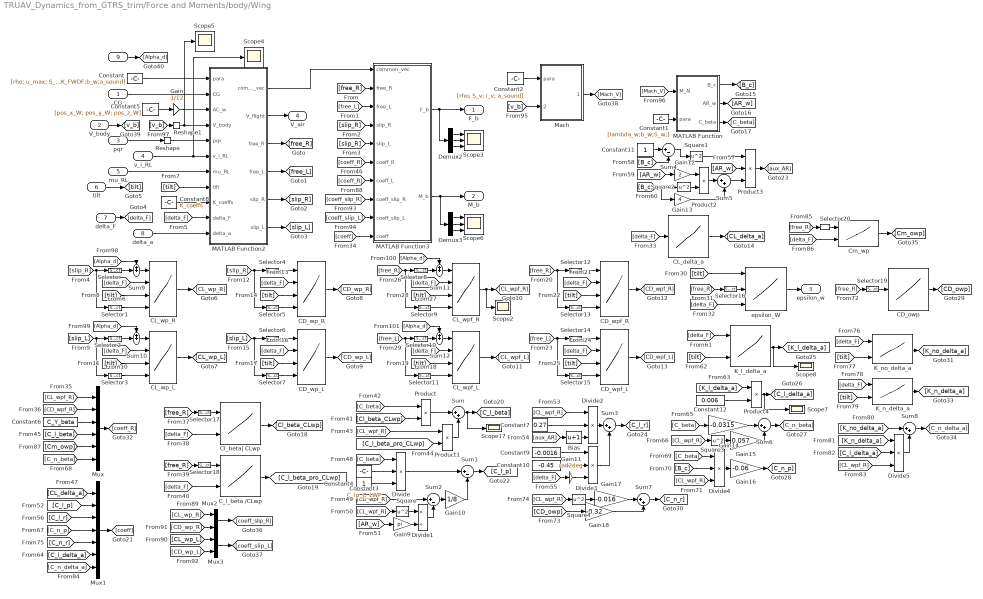
== system TRUAV_Dynamics_from_GTRS_trim/Force and Moments/body/Wing ==
  CG : Inport
  V_body : Inport  Port=2
  pqr : Inport  Port=3
  v_i_RL : Inport  Port=4
  mu_RL : Inport  Port=5
  tilt : Inport  Port=6
  delta_F : Inport  Port=7
  delta_a : Inport  Port=8
  " " : Inport  Port=9
  Bias : Bias  Bias=1  SaturateOnIntegerOverflow=off
  CD_owp : Lookup_n-D  NumberOfTableDimensions=1  BreakpointsForDimension1=Mach_brk  BreakpointsForDimension2=beta_m_rad_cn  BreakpointsForDimension3=beta_m_rad  BreakpointsForDimension4=mach_vec  Table=CD0_high_Mach_data  InternalRulePriority=Speed  RndMeth=Simplest
  CD_wp_L : Lookup_n-D  NumberOfTableDimensions=4  BreakpointsForDimension1=alpha_WS_CL_rad  BreakpointsForDimension2=flap_rad  BreakpointsForDimension3=beta_m_WS_CL_rad  BreakpointsForDimension4=mach_WS_vec  Table=CD_4D_table  InternalRulePriority=Speed  RndMeth=Simplest
      settings: InputPortMap=u0,u1,u2,u3
  CD_wp_R : Lookup_n-D  NumberOfTableDimensions=4  BreakpointsForDimension1=alpha_WS_CL_rad  BreakpointsForDimension2=flap_rad  BreakpointsForDimension3=beta_m_WS_CL_rad  BreakpointsForDimension4=mach_WS_vec  Table=CD_4D_table  InternalRulePriority=Speed  RndMeth=Simplest
      settings: InputPortMap=u0,u1,u2,u3
  CD_wpf_L : Lookup_n-D  NumberOfTableDimensions=4  BreakpointsForDimension1=alpha_WS_CL_rad  BreakpointsForDimension2=flap_rad  BreakpointsForDimension3=beta_m_WS_CL_rad  BreakpointsForDimension4=mach_WS_vec  Table=CD_4D_table  InternalRulePriority=Speed  RndMeth=Simplest
      settings: InputPortMap=u0,u1,u2,u3
  CD_wpf_R : Lookup_n-D  NumberOfTableDimensions=4  BreakpointsForDimension1=alpha_WS_CL_rad  BreakpointsForDimension2=flap_rad  BreakpointsForDimension3=beta_m_WS_CL_rad  BreakpointsForDimension4=mach_WS_vec  Table=CD_4D_table  InternalRulePriority=Speed  RndMeth=Simplest
      settings: InputPortMap=u0,u1,u2,u3
  CL_delta_a : Lookup_n-D  NumberOfTableDimensions=1  BreakpointsForDimension1=flap_rad  BreakpointsForDimension2=flap_rad  BreakpointsForDimension3=beta_m_rad  BreakpointsForDimension4=mach_vec  Table=C_L_delta_a_table  InternalRulePriority=Speed  RndMeth=Simplest
  CL_wp_L : Lookup_n-D  NumberOfTableDimensions=4  BreakpointsForDimension1=alpha_WS_CL_rad  BreakpointsForDimension2=flap_rad  BreakpointsForDimension3=beta_m_WS_CL_rad  BreakpointsForDimension4=mach_WS_vec  Table=CL_4D_table  InternalRulePriority=Speed  RndMeth=Simplest
      settings: InputPortMap=u0,u1,u2,u3
  CL_wp_R : Lookup_n-D  NumberOfTableDimensions=4  BreakpointsForDimension1=alpha_WS_CL_rad  BreakpointsForDimension2=flap_rad  BreakpointsForDimension3=beta_m_WS_CL_rad  BreakpointsForDimension4=mach_WS_vec  Table=CL_4D_table  InternalRulePriority=Speed  RndMeth=Simplest
      settings: InputPortMap=u0,u1,u2,u3
  CL_wpf_L : Lookup_n-D  NumberOfTableDimensions=4  BreakpointsForDimension1=alpha_WS_CL_rad  BreakpointsForDimension2=flap_rad  BreakpointsForDimension3=beta_m_WS_CL_rad  BreakpointsForDimension4=mach_WS_vec  Table=CL_4D_table  InternalRulePriority=Speed  RndMeth=Simplest
      settings: InputPortMap=u0,u1,u2,u3
  CL_wpf_R : Lookup_n-D  NumberOfTableDimensions=4  BreakpointsForDimension1=alpha_WS_CL_rad  BreakpointsForDimension2=flap_rad  BreakpointsForDimension3=beta_m_WS_CL_rad  BreakpointsForDimension4=mach_WS_vec  Table=CL_4D_table  InternalRulePriority=Speed  RndMeth=Simplest
      settings: InputPortMap=u0,u1,u2,u3
  C_l_beta /CLwp : Lookup_n-D  BreakpointsForDimension1=beta_WF_Cl_rad  BreakpointsForDimension2=flap_rad  BreakpointsForDimension3=beta_m_rad  BreakpointsForDimension4=mach_vec  Table=C_l_beta_pro_CLwp_table  InternalRulePriority=Speed  RndMeth=Simplest
      settings: InputPortMap=u0,u1
  Cl_beta| CLwp : Lookup_n-D  BreakpointsForDimension1=beta_WF_Cl_rad  BreakpointsForDimension2=flap_rad  BreakpointsForDimension3=beta_m_rad  BreakpointsForDimension4=mach_vec  Table=C_l_beta_CLwp_table  InternalRulePriority=Speed  RndMeth=Simplest
      settings: InputPortMap=u0,u1
  Cm_wp : Lookup_n-D  BreakpointsForDimension1=beta_WF_CL_rad  BreakpointsForDimension2=flap_rad  BreakpointsForDimension3=beta_m_rad  BreakpointsForDimension4=mach_vec  Table=C_m_wp_table  InternalRulePriority=Speed  RndMeth=Simplest
      settings: InputPortMap=u0,u1
  Constant : Constant  Value=[rho; u_max; S_max;S_w;i_w;c_w;K_FWO;K_FWDF;b_w;a_sound]
  Constant1 : Constant  Value=[lambda_w;b_w;S_w;]
  Constant10 : Constant  Value=-0.45
  Constant11 : Constant
  Constant12 : Constant  Value=0.006
  Constant2 : Constant  Value=[rho; S_v; i_v; a_sound]
  Constant3 : Constant  Value=C_lp_C_LWP
  Constant4 : Constant
  Constant5 : Constant  Value=[pos_x_W; pos_y_W; pos_z_W]
  Constant6 : Constant  Value=C_Y_beta
  Constant7 : Constant  Value=0.27
  Constant8 : Constant  Value=K_coeffs
  Constant9 : Constant  Value=-0.0016
  Demux2 : Demux  Outputs=3
  Demux3 : Demux  Outputs=3
  Divide{,2..5} (5 alike) : Product  Inputs=***
  Divide1 : Product  Inputs=*/
  Gain : Gain  Gain=1/12
  Gain10 : Gain  Gain=1/8
  Gain11 : Gain  Gain=rad2deg
  Gain12 : Gain  Gain=2
  Gain13 : Gain  Gain=4
  Gain14 : Gain  Gain=-0.0315
  Gain15 : Gain  Gain=0.057
  Gain16 : Gain  Gain=-0.06
  Gain17 : Gain  Gain=-0.016
  Gain18 : Gain  Gain=-0.32
  Gain9 : Gain  Gain=pi
  K_l_delta_a : Lookup_n-D  BreakpointsForDimension1=flap_rad  BreakpointsForDimension2=mast_rad  BreakpointsForDimension3=beta_m_rad  BreakpointsForDimension4=mach_vec  Table=K1delta_data  InternalRulePriority=Speed  RndMeth=Simplest
      settings: InputPortMap=u0,u1
  K_n_delta_a : Lookup_n-D  BreakpointsForDimension1=flap_rad  BreakpointsForDimension2=beta_m_rad_cn  BreakpointsForDimension3=beta_m_rad  BreakpointsForDimension4=mach_vec  Table=Kn_delta_data  InternalRulePriority=Speed  RndMeth=Simplest
      settings: InputPortMap=u0,u1
  K_no_delta_a : Lookup_n-D  BreakpointsForDimension1=flap_rad  BreakpointsForDimension2=beta_m_rad_cn  BreakpointsForDimension3=beta_m_rad  BreakpointsForDimension4=mach_vec  Table=Kno_delta_data  InternalRulePriority=Speed  RndMeth=Simplest
      settings: InputPortMap=u0,u1
  MATLAB Function : MATLAB Function  TreatAsAtomicUnit=on
  MATLAB Function2 : MATLAB Function  TreatAsAtomicUnit=on
  MATLAB Function3 : MATLAB Function  TreatAsAtomicUnit=on
  Mach : MATLAB Function  TreatAsAtomicUnit=on
  Mux : Mux  Inputs=6
  Mux1 : Mux  Inputs=7
  Mux2 : Mux  Inputs=2
  Mux3 : Mux  Inputs=2
  Product{,1..2,4} (4 alike) : Product
  Product3 : Product  Inputs=3
  Reshape : Reshape  OutputDimensionality=Column vector (2-D)
  Reshape1 : Reshape  OutputDimensionality=Column vector (2-D)
  Scope{2,4..5,7..8,17} (6 alike) : Scope
  Scope3 : Scope  NumInputPorts=3
  Scope6 : Scope  NumInputPorts=3
  Selector{,2,4,6} (4 alike) : Selector  InputPortWidth=4  IndexOptions=Index vector (dialog)  Indices=[1]  OutputSizes=1
  Selector{1,3,5,7} (4 alike) : Selector  InputPortWidth=4  IndexOptions=Index vector (dialog)  Indices=[4]  OutputSizes=1
  Selector{8,10,12,14,16} (5 alike) : Selector  InputPortWidth=12  IndexOptions=Index vector (dialog)  Indices=[1]  OutputSizes=1
  Selector{9,11,13,15,19..20} (6 alike) : Selector  InputPortWidth=12  IndexOptions=Index vector (dialog)  Indices=[3]  OutputSizes=1
  Selector17 : Selector  InputPortWidth=12  IndexOptions=Index vector (dialog)  Indices=[9]  OutputSizes=1
  Selector18 : Selector  InputPortWidth=12  IndexOptions=Index vector (dialog)  Indices=[9]  OutputSizes=1
  Square{,1..4} (5 alike) : Math  Operator=square
  Sum{,3,5..8} (6 alike) : Sum  Inputs=|++
  Sum1 : Sum  Inputs=|+-
  Sum{9..12} (4 alike) : Sum  Inputs=++|
  Sum2 : Sum  Inputs=|+-
  Sum4 : Sum  Inputs=|+-
  epsilon_W : Lookup_n-D  NumberOfTableDimensions=3  BreakpointsForDimension1=beta_m_epsilon_M_rad  BreakpointsForDimension2=alpha_WF_epsilon_M_rad  BreakpointsForDimension3=flap_rad  BreakpointsForDimension4=mach_vec  Table=epsilon_W_table  InternalRulePriority=Speed  RndMeth=Simplest
      settings: InputPortMap=u0,u1,u2
  F_b : Outport
  M_b : Outport  Port=2
  epsilon_w : Outport  Port=3
  V_air : Outport  Port=4
  wires:
  Constant8/1 -> MATLAB Function2/9(K_coeffs)
  mu_RL/1 -> MATLAB Function2/7(mu_RL)
  Constant5/1 -> Gain/1
  Constant/1 -> MATLAB Function2/1(para)
  Gain/1 -> MATLAB Function2/3(AC_w)
  tilt/1 -> [tilt]
  [v_b] -> Reshape1/1
  v_i_RL/1 -> Scope4/1, MATLAB Function2/6(v_i_RL)
  pqr/1 -> Reshape/1
  CG/1 -> MATLAB Function2/2(CG)
  delta_a/1 -> MATLAB Function2/11(delta_a)
  Constant1/1 -> MATLAB Function/2(para)
  MATLAB Function2/1(common_vec) -> MATLAB Function3/1(common_vec)
  MATLAB Function2/3(free_R) -> [free_R]
  [free_R] -> MATLAB Function3/2(free_R)
  MATLAB Function2/6(slip_L) -> [slip_L]
  MATLAB Function2/5(slip_R) -> [slip_R]
  MATLAB Function2/4(free_L) -> [free_L]
  [free_L] -> MATLAB Function3/3(free_L)
  [slip_R] -> MATLAB Function3/4(slip_R)
  [slip_R] -> MATLAB Function3/5(slip_L)
  Cm_wp/1 -> [Cm_owp]
  K_l_delta_a/1 -> Scope8/1, [K_l_delta_a]
  epsilon_W/1 -> epsilon_w/1
  [slip_R] -> Selector1/1, Selector/1
  Selector/1 -> Sum9/2
  delta_F/1 -> [delta_F]
  [delta_F] -> MATLAB Function2/10(delta_F)
  [delta_F] -> CL_wp_R/2
  [tilt] -> MATLAB Function2/8(tilt)
  Selector1/1 -> CL_wp_R/4
  [tilt] -> CL_wp_R/3
  CL_wp_R/1 -> [CL_wp_R]
  CL_wp_L/1 -> [CL_wp_L]
  [slip_L] -> Selector3/1, Selector2/1
  [tilt] -> CL_wp_L/3
  Selector3/1 -> CL_wp_L/4
  Selector2/1 -> Sum10/2
  [delta_F] -> CL_wp_L/2
  [slip_R] -> Selector5/1, Selector4/1
  [tilt] -> CD_wp_R/3
  Selector5/1 -> CD_wp_R/4
  Selector4/1 -> CD_wp_R/1
  [delta_F] -> CD_wp_R/2
  CD_wp_R/1 -> [CD_wp_R]
  CD_wp_L/1 -> [CD_wp_L]
  [delta_F] -> CD_wp_L/2
  Selector6/1 -> CD_wp_L/1
  Selector7/1 -> CD_wp_L/4
  [tilt] -> CD_wp_L/3
  [slip_L] -> Selector6/1, Selector7/1
  [free_L] -> Selector15/1, Selector14/1
  [tilt] -> CD_wpf_L/3
  Selector15/1 -> CD_wpf_L/4
  Selector14/1 -> CD_wpf_L/1
  [delta_F] -> CD_wpf_L/2
  CD_wpf_L/1 -> [CD_wpf_L]
  CD_wpf_R/1 -> [CD_wpf_R]
  [delta_F] -> CD_wpf_R/2
  Selector12/1 -> CD_wpf_R/1
  Selector13/1 -> CD_wpf_R/4
  [tilt] -> CD_wpf_R/3
  [free_R] -> Selector12/1, Selector13/1
  [delta_F] -> CL_wpf_L/2
  Selector10/1 -> Sum12/2
  Selector11/1 -> CL_wpf_L/4
  [tilt] -> CL_wpf_L/3
  [free_L] -> Selector10/1, Selector11/1
  CL_wpf_L/1 -> [CL_wpf_L]
  CL_wpf_R/1 -> Scope2/1, [CL_wpf_R]
  [tilt] -> CL_wpf_R/3
  Selector9/1 -> CL_wpf_R/4
  [delta_F] -> CL_wpf_R/2
  Selector8/1 -> Sum11/2
  [free_R] -> Selector8/1, Selector9/1
  [tilt] -> epsilon_W/1
  [free_R] -> Selector16/1
  Selector16/1 -> epsilon_W/2
  [delta_F] -> epsilon_W/3
  [delta_F] -> CL_delta_a/1
  CL_delta_a/1 -> [CL_delta_a]
  [coeff] -> MATLAB Function3/10(coeff)
  MATLAB Function/1(B_c) -> [B_c]
  MATLAB Function/2(AR_w) -> [AR_w]
  MATLAB Function/3(C_beta) -> [C_beta]
  [free_R] -> Selector17/1
  Selector17/1 -> Cl_beta| CLwp/1
  [delta_F] -> Cl_beta| CLwp/2
  Cl_beta| CLwp/1 -> [Cl_beta_CLwp]
  [free_R] -> Selector18/1
  Selector18/1 -> C_l_beta /CLwp/1
  [delta_F] -> C_l_beta /CLwp/2
  C_l_beta /CLwp/1 -> [C_l_beta_pro_CLwp]
  [Cl_beta_CLwp] -> Product/2
  [C_beta] -> Product/1
  Product/1 -> Sum/1
  Sum/1 -> Scope17/1, [C_l_beta]
  [CL_wpf_R] -> Product1/1
  [C_l_beta_pro_CLwp] -> Product1/2
  Product1/1 -> Sum/2
  [CL_wpf_R] -> Mux/1
  [CD_wpf_R] -> Mux/2
  Constant6/1 -> Mux/3
  [C_l_beta] -> Mux/4
  [coeff_R] -> MATLAB Function3/6(coeff_R)
  [CL_delta_a] -> Mux1/1
  Mux1/1 -> [coeff]
  [C_l_r] -> Mux1/3
  [C_beta] -> Divide/1
  Constant3/1 -> Divide/2
  Constant4/1 -> Divide/3
  Divide/1 -> Sum1/1
  [CL_wpf_R] -> Square/1
  Square/1 -> Divide1/1
  Gain9/1 -> Divide1/2
  [AR_w] -> Gain9/1
  [CD_wpf_R] -> Sum2/1
  Divide1/1 -> Sum2/2
  Sum2/1 -> Gain10/1
  Gain10/1 -> Sum1/2
  Sum1/1 -> [C_l_p]
  [C_l_p] -> Mux1/2
  [aux_AR] -> Bias/1
  Bias/1 -> Divide2/3
  Constant7/1 -> Divide2/2
  [CL_wpf_R] -> Divide2/1
  Constant9/1 -> Divide3/1
  Constant10/1 -> Divide3/2
  [delta_F] -> Gain11/1
  Gain11/1 -> Divide3/3
  Divide2/1 -> Sum3/1
  Divide3/1 -> Sum3/2
  Sum3/1 -> [C_l_r]
  Constant11/1 -> Sum4/1
  [B_c] -> Sum4/2
  Sum4/1 -> Square1/1
  [B_c] -> Gain13/1, Square2/1
  [AR_w] -> Gain12/1
  Gain12/1 -> Product2/1
  Square2/1 -> Product2/2
  Product2/1 -> Sum5/1
  Gain13/1 -> Sum5/2
  Sum5/1 -> Product3/3
  Square1/1 -> Product3/1
  [AR_w] -> Product3/2
  Product3/1 -> [aux_AR]
  [delta_F] -> K_l_delta_a/1
  [tilt] -> K_l_delta_a/2
  [K_l_delta_a] -> Product4/1
  Constant12/1 -> Product4/2
  Product4/1 -> Scope7/1, [C_l_delta_a]
  [C_l_delta_a] -> Mux1/6
  [C_beta] -> Gain14/1
  [CL_wpf_R] -> Square3/1
  Square3/1 -> Gain15/1
  Gain14/1 -> Sum6/1
  Gain15/1 -> Sum6/2
  Sum6/1 -> [C_n_beta]
  [C_n_p] -> Mux1/4
  [C_n_beta] -> Mux/6
  [CL_wpf_R] -> Divide4/3
  Divide4/1 -> Gain16/1
  [B_c] -> Divide4/2
  [C_beta] -> Divide4/1
  Gain16/1 -> [C_n_p]
  [free_R] -> Selector19/1
  Selector19/1 -> CD_owp/1
  CD_owp/1 -> [CD_owp]
  [CL_wpf_R] -> Square4/1
  Square4/1 -> Gain17/1
  Gain17/1 -> Sum7/1
  [CD_owp] -> Gain18/1
  Gain18/1 -> Sum7/2
  Sum7/1 -> [C_n_r]
  [C_n_r] -> Mux1/5
  [tilt] -> K_no_delta_a/2
  [delta_F] -> K_no_delta_a/1
  K_no_delta_a/1 -> [K_no_delta_a]
  Mux/1 -> [coeff_R]
  [tilt] -> K_n_delta_a/2
  [delta_F] -> K_n_delta_a/1
  K_n_delta_a/1 -> [K_n_delta_a]
  [K_n_delta_a] -> Divide5/1
  [C_l_delta_a] -> Divide5/2
  [CL_wpf_R] -> Divide5/3
  [K_no_delta_a] -> Sum8/1
  Divide5/1 -> Sum8/2
  Sum8/1 -> [C_n_delta_a]
  [C_n_delta_a] -> Mux1/7
  [free_R] -> Selector20/1
  Selector20/1 -> Cm_wp/1
  [delta_F] -> Cm_wp/2
  [Cm_owp] -> Mux/5
  [coeff_R] -> MATLAB Function3/7(coeff_L)
  [CL_wp_R] -> Mux2/1
  [CD_wp_R] -> Mux2/2
  [CL_wp_L] -> Mux3/1
  [CD_wp_L] -> Mux3/2
  Mux2/1 -> [coeff_slip_R]
  Mux3/1 -> [coeff_slip_L]
  [coeff_slip_R] -> MATLAB Function3/8(coeff_slip_R)
  [coeff_slip_L] -> MATLAB Function3/9(coeff_slip_L)
  MATLAB Function2/2(V_flight) -> V_air/1
  [v_b] -> Mach/2(V_body)
  Mach/1(Mach_N) -> [Mach_V]
  Constant2/1 -> Mach/1(para)
  [Mach_V] -> MATLAB Function/1(M_N)
  Reshape/1 -> MATLAB Function2/5(pqr)
  Reshape1/1 -> Scope5/1, MATLAB Function2/4(V_body)
  MATLAB Function3/1(F_b) -> Demux2/1, F_b/1
  Demux2/2 -> Scope3/2
  Demux2/1 -> Scope3/1
  Demux2/3 -> Scope3/3
  MATLAB Function3/2(M_b) -> Demux3/1, M_b/1
  Demux3/2 -> Scope6/2
  Demux3/1 -> Scope6/1
  Demux3/3 -> Scope6/3
  V_body/1 -> [v_b]
  " "/1 -> [Alpha_d]
  Sum9/1 -> CL_wp_R/1
  [Alpha_d] -> Sum9/1
  [Alpha_d] -> Sum10/1
  Sum10/1 -> CL_wp_L/1
  Sum11/1 -> CL_wpf_R/1
  [Alpha_d] -> Sum11/1
  Sum12/1 -> CL_wpf_L/1
  [Alpha_d] -> Sum12/1

== matlab function TRUAV_Dynamics_from_GTRS_trim/Force and Moments/Propulsion1/Rotor Assembly 1 Right/计算挥舞角、桨尖马赫数 桨叶升力线斜率1 ==
  data: para input; V input; beta_F_Para output; r_n input; tilt input; mu input; AB input; alpha input; pqr input; v_1d input; M_tip output; a_MR output; lamda input
function [beta_F_Para, M_tip, a_MR] = rotor_cal1(...
    para, V, r_n, tilt, mu, AB, alpha, pqr, v_1d, lamda)
% 整合旋翼气动与挥舞计算模型（包含洛克数自动计算）
% 输入：
%   para     - 参数向量 [R, theta_0_W, theta_0_R, theta_twist, a_sound, alpha_0, rho, c, I_b]
%              R: 旋翼半径 [ft]
%              theta_0_W: 悬停总距 [rad]（对应β_M=0）
%              theta_0_R: 悬停总距 [rad]（对应β_M=90°）
%              theta_twist: 桨叶线性扭转率 [rad]
%              a_sound: 当地声速 [ft/s]
%              alpha_0: 桨叶零升迎角修正 [rad]
%              rho: 空气密度 [slug/ft³]
%              c: 桨叶弦长 [in]（自动转换为ft）
%              I_b: 桨叶挥舞惯性矩 [slug·ft²]
%   V        - 飞机前进速度 [ft/s]
%   r_n      - 展向位置比率（通常为1，代表桨尖）
%   tilt   - 短舱倾角 [rad]
%   mu       - 前进比（无量纲）
%   AB       - 周期变距向量 [A1, B1]  [rad]
%   alpha    - 迎角[rad]
%   gamma_b  - 洛克数（占位符，实际会被覆盖计算，可任意值）
%   pqr      - 机体角速度 [p,q,r] [rad/s]
%   lamda    - 入流比（未使用，保留接口）
%   Psi    - 方位角 [rad]
% 输出：
%   beta_F     - 挥舞角 [rad]
%   M_tip    - 桨尖马赫数
%   a_MR     - 旋翼升力线斜率 [1/rad]

% 解析参数
R = para(1);
theta_0_W = para(2);
theta_0_R = para(3);
theta_twist = para(4);
a_sound = para(5);
alpha_0 = para(6);
rho = para(7);
c = para(8);
I_b = para(9);

p = pqr(1);
q = pqr(2);
A1 = AB(2);
B1 = AB(3);

% ========== 1. 计算桨尖马赫数 M_tip ==========
V_tip = sqrt(V^2 + (r_n*R)^2 + 2*V*r_n*R*cos(tilt));
M_tip = V_tip / a_sound;

% ========== 2. 计算升力线斜率 a_MR（Kleinhesselink 论文）==========
denom = sqrt(1 - (0.75*M_tip)^2 * sin(tilt));
if denom < 1e-6
    denom = 1e-6;
end
 a_MR = (4.95 + mu * (8 + 30*mu)) / denom;

% ========== 3. 计算洛克数 gamma ==========
gamma_b_calc = rho * a_MR * c * R^4 / I_b;   % 无量纲洛克数

% ========== 4. 计算挥舞角 ==========
theta0 = 2*(tilt)/pi * (theta_0_W - theta_0_R) + theta_0_R;
alpha_s = alpha - tilt;

% 4.1 后倒角 a1s（纵向挥舞）
term1 = (2*mu) / (1 - 0.5*mu^2);
term2 = (4/3)*theta0 + theta_twist + mu*alpha_s - v_1d/(r_n*R);
term3 = - (1 + 1.5*mu^2) / (1 - 0.5*mu^2) * B1;
term4 = -16/gamma_b_calc * q / r_n + p / r_n;
a1s = term1 * term2 + term3 + term4/(1 - 0.5*mu^2);

% 4.2 侧倒角 b1s（横向挥舞）
term1_b = (2*mu) / (1 + 0.5*mu^2);
term2_b = (4/3) * mu * alpha_0;
term3_b = A1;
term4_b = -16/gamma_b_calc * p / r_n;
term5_b = - q / r_n;
b1s = term1_b * term2_b + term3_b + (term4_b + term5_b)/(1 + 0.5*mu^2);

% 锥度角 a0（简化）
gamma_used = gamma_b_calc;   % 使用计算得到的洛克数
a0 = (gamma_used/8) * ((4/3)*theta0*(1 + mu^2) + 2*lamda*mu);

% 挥舞角随方位角变化
beta_F_Para = [a0 a1s b1s];

end

== matlab function TRUAV_Dynamics_from_GTRS_trim/6DOF Model/disturbance2/Disturb1 ==
  data: t input; y output
function y = fcn(t)
    y=0.5+1.5*cos(0.1*pi*t);

end

== matlab function TRUAV_Dynamics_from_GTRS_trim/6DOF Model/disturbance2/Disturb4 ==
  data: t input; y output
function y = fcn(t)
    y=1+2*sin(0.05*pi*t);
    
end

== matlab function TRUAV_Dynamics_from_GTRS_trim/6DOF Model/disturbance2/Disturb2 ==
  data: t input; y output
function y = fcn(t)
    y=-1+2*sin(0.1*pi*t);
%     if t>=8&&t<=14
%         y=y1*(1+sin(1/6*pi*(t-8)));
%     elseif t>=21&&t<=23
%         y=y1*(1+sin(1/2*pi*(t-21)));
%     else 
%         y=y1;
%     end
end
